simulink model "untitled1"  (R2023b)
settings: Solver=VariableStepAuto  StartTime=0.0  StopTime=10  RelTol=1e-3
undefined symbols (not defined in the file): magnitude
libraries: dspfdesign x2
settings Model: Creator=mrabd  LastModifiedBy=mrabd

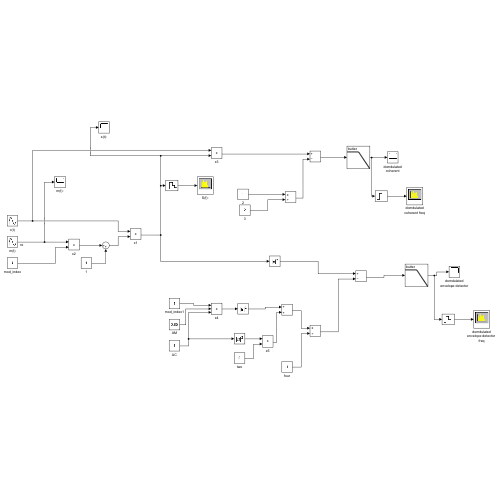
[thumbnail: Simulink's stored preview of the top-level diagram]
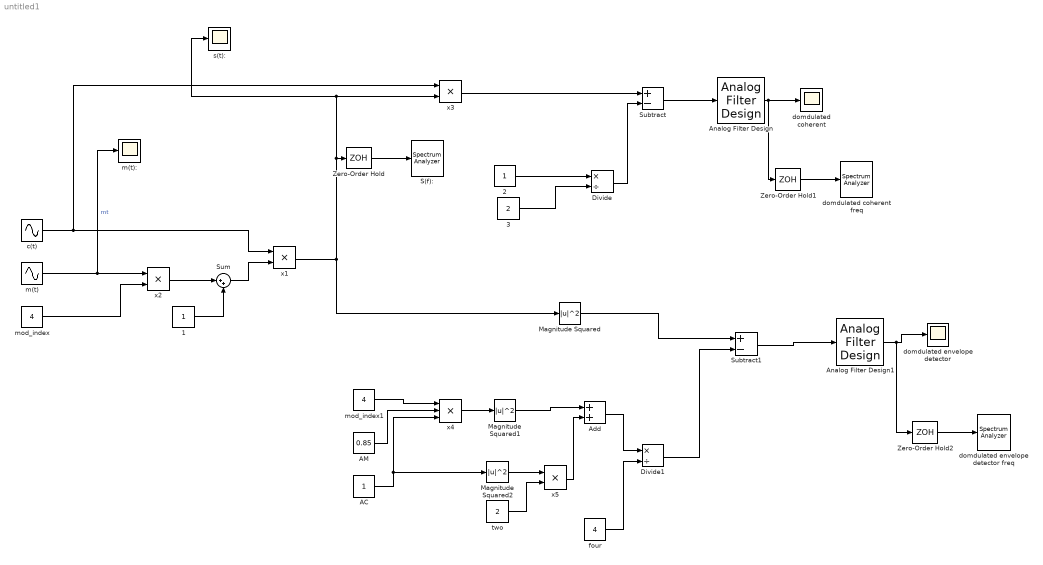
== system untitled1 ==
  1 : Constant
  2 : Constant
  3 : Constant  Value=2
  AC : Constant
  AM : Constant  Value=0.85
  Add : Sum
  Analog Filter Design : dspfdesign/Analog Filter Design  method=Butterworth  filttype=Lowpass  N=8  Wlo=50000  Whi=80  Rp=2  Rs=40
  Analog Filter Design1 : dspfdesign/Analog Filter Design  method=Butterworth  filttype=Lowpass  N=8  Wlo=50000  Whi=80  Rp=2  Rs=40
  Divide : Product  Inputs=*/
  Divide1 : Product  Inputs=*/
  Magnitude Squared : Math  Operator=magnitude^2
  Magnitude Squared1 : Math  Operator=magnitude^2
  Magnitude Squared2 : Math  Operator=magnitude^2
  S(f): : SpectrumAnalyzer  WindowPosition=[770.000000,454.000000,766.000000,381.000000,]  ScopeFrameLocation=window  SampleRateSource=Property  SampleRate=44.1e3  PlotAsTwoSidedSpectrum=off  FrequencyScale=Log  FrequencySpan=Start and stop frequencies  StartFrequency=20  StopFrequency=20e3  YLimits=[-167.38383736,53.70784644]
  Subtract : Sum  Inputs=+-
  Subtract1 : Sum  Inputs=+-
  Sum : Sum  Inputs=|++
  Zero-Order Hold : ZeroOrderHold  SampleTime=-1
  Zero-Order Hold1 : ZeroOrderHold  SampleTime=-1
  Zero-Order Hold2 : ZeroOrderHold  SampleTime=-1
  c(t) : Sin  Frequency=94200  SampleTime=0
  domdulated coherent : Scope
  domdulated coherent freq : SpectrumAnalyzer  WindowPosition=[2.000000,42.000000,766.000000,793.000000,]  ScopeFrameLocation=window  SampleRateSource=Property  SampleRate=44.1e3  PlotAsTwoSidedSpectrum=off  FrequencyScale=Log  FrequencySpan=Start and stop frequencies  StartFrequency=20  StopFrequency=20e3  YLimits=[-188.84923885,56.05767269]
  domdulated envelope detector : Scope
  domdulated envelope detector freq : SpectrumAnalyzer  WindowPosition=[770.000000,42.000000,766.000000,381.000000,]  ScopeFrameLocation=window  SampleRateSource=Property  SampleRate=44.1e3  PlotAsTwoSidedSpectrum=off  FrequencyScale=Log  FrequencySpan=Start and stop frequencies  StartFrequency=20  StopFrequency=20e3  YLimits=[-179.21743978,61.67702887]  SelectedToolstripTab=spectrumAnalyzerToolstrip.estimationTab
  four : Constant  Value=4
  m(t) : Sin  Amplitude=0.85  Frequency=6280  SampleTime=0
  m(t): : Scope
  mod_index : Constant  Value=4
  mod_index1 : Constant  Value=4
  s(t): : Scope
  two : Constant  Value=2
  x{1..3,5} (4 alike) : Product
  x4 : Product  Inputs=3
  wires:
  m(t)/1 -> m(t):/1, x2/1  "mt"
  mod_index/1 -> x2/2
  x2/1 -> Sum/1
  1/1 -> Sum/2
  c(t)/1 -> x3/1, x1/1
  Sum/1 -> x1/2
  Zero-Order Hold/1 -> S(f):/1
  Divide/1 -> Subtract/2
  x3/1 -> Subtract/1
  2/1 -> Divide/1
  3/1 -> Divide/2
  Subtract/1 -> Analog Filter Design/1
  x1/1 -> s(t):/1, x3/2, Zero-Order Hold/1, Magnitude Squared/1
  mod_index1/1 -> x4/1
  AM/1 -> x4/2
  AC/1 -> Magnitude Squared2/1, x4/3
  x4/1 -> Magnitude Squared1/1
  Magnitude Squared2/1 -> x5/1
  two/1 -> x5/2
  Magnitude Squared1/1 -> Add/1
  x5/1 -> Add/2
  four/1 -> Divide1/2
  Add/1 -> Divide1/1
  Magnitude Squared/1 -> Subtract1/1
  Divide1/1 -> Subtract1/2
  Subtract1/1 -> Analog Filter Design1/1
  Analog Filter Design1/1 -> Zero-Order Hold2/1, domdulated envelope detector/1
  Zero-Order Hold1/1 -> domdulated coherent freq/1
  Analog Filter Design/1 -> Zero-Order Hold1/1, domdulated coherent/1
  Zero-Order Hold2/1 -> domdulated envelope detector freq/1
